simulink subsystem "gyroscope"  (R2023b)
settings: Solver=VariableStepAuto  StartTime=0.0  StopTime=10.0  RelTol=1e-3
undefined symbols (not defined in the file or in its folder): IMU
libraries: sensors_subsystems x5, simulink_extras x2
settings Model: Creator=brent  LastModifiedBy=brent

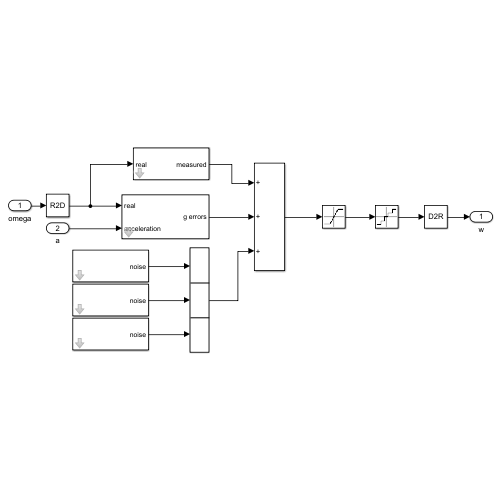
[thumbnail: Simulink's stored preview of the top-level diagram]
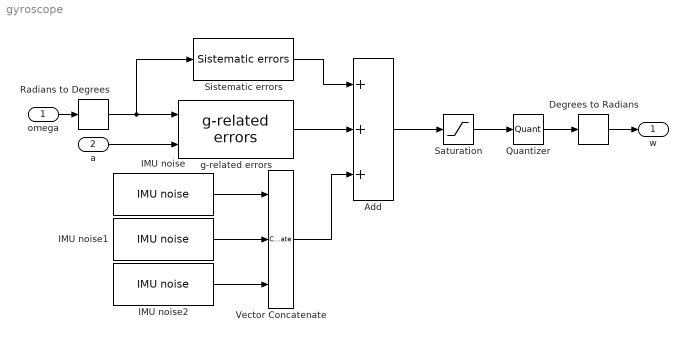
== system gyroscope ==
  omega : Inport
  a : Inport  Port=2
  Add : Sum  Inputs=+++
  Degrees to Radians : simulink_extras/Transformations/Degrees to Radians
  IMU noise : sensors_subsystems/IMU noise  data=IMU.gyroscope  arw_seed=abs(round(randn(1)*1e4))  bi_seed=abs(round(randn(1)*1e4))
      settings: SourceProductName=Sensors library
  IMU noise1 : sensors_subsystems/IMU noise  data=IMU.gyroscope  arw_seed=abs(round(randn(1)*1e4))  bi_seed=abs(round(randn(1)*1e4))
      settings: SourceProductName=Sensors library
  IMU noise2 : sensors_subsystems/IMU noise  data=IMU.gyroscope  arw_seed=abs(round(randn(1)*1e4))  bi_seed=abs(round(randn(1)*1e4))
      settings: SourceProductName=Sensors library
  Quantizer : Quantizer  QuantizationInterval=IMU.gyroscope.resolution.value
  Radians to Degrees : simulink_extras/Transformations/Radians to Degrees
  Saturation : Saturate  UpperLimit=IMU.gyroscope.range.value  LowerLimit=-IMU.gyroscope.range.value
  Sistematic errors : sensors_subsystems/Sistematic errors  data=IMU.gyroscope
      settings: SourceProductName=Sensors library
  Vector Concatenate : Concatenate  NumInputs=3
  g-related errors : sensors_subsystems/g-related errors  gyro=IMU.gyroscope
      settings: SourceProductName=Sensors library
  w : Outport
  wires:
  a/1 -> g-related errors/2
  omega/1 -> Radians to Degrees/1
  Radians to Degrees/1 -> Sistematic errors/1, g-related errors/1
  g-related errors/1 -> Add/2
  Sistematic errors/1 -> Add/1
  Add/1 -> Saturation/1
  Saturation/1 -> Quantizer/1
  Quantizer/1 -> Degrees to Radians/1
  Degrees to Radians/1 -> w/1
  IMU noise/1 -> Vector Concatenate/1
  IMU noise2/1 -> Vector Concatenate/3
  IMU noise1/1 -> Vector Concatenate/2
  Vector Concatenate/1 -> Add/3
